simulink model "quadrotor"  (R2020a)
settings: Solver=ode4  StartTime=0.0  StopTime=10  FixedStep=0.01  RelTol=1e-3  EnableMultiTasking=on
settings Model: Creator=fmina  LastModifiedBy=Chenhao
settings DataIOCC: ReturnWorkspaceOutputs=off
settings OptimizationCC: LifeSpan=inf
settings DebuggingCC: SFUnexpectedBacktrackingDiag=warning  SFNoUnconditionalDefaultTransitionDiag=warning  SFExecutionAtInitializationDiag=none  ArithmeticOperatorsInVariantConditions=warning
settings SFSimCC: SimUseLocalCustomCode=off  CustomCodeUndefinedFunction=UseInterfaceOnly
settings RTWCC: RTWUseLocalCustomCode=off
settings CodeAppCC: StateflowObjectComments=on
settings GRTTargetCC: TargetLangStandard=C89/C90 (ANSI)
settings ConfigComp: CovMetricSettings=dw  CovHtmlReporting=on  CovSaveCumulativeToWorkspaceVar=on  CovSaveSingleToWorkspaceVar=on  CovExternalEMLEnable=off

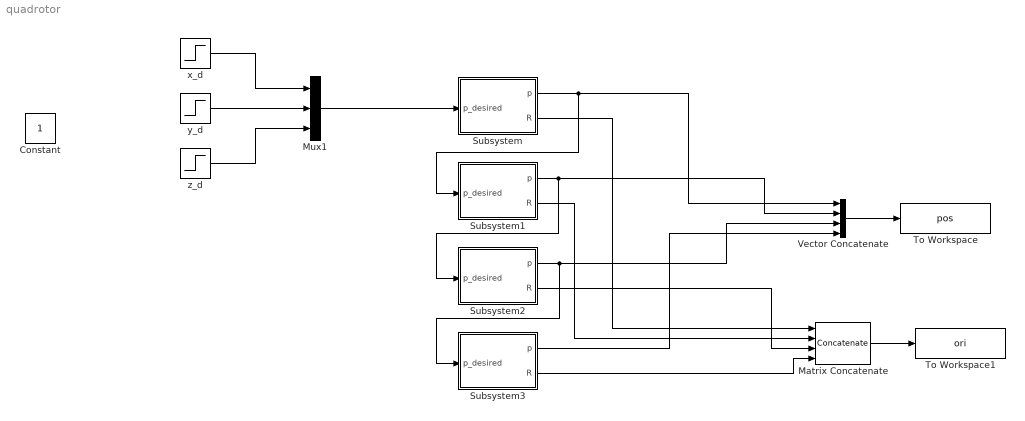
== system quadrotor ==
  Matrix Concatenate : Concatenate  NumInputs=4  Mode=Multidimensional array  ConcatenateDimension=2
  Mux1 : Mux  Inputs=3
  Subsystem : Subsystem
  Subsystem1 : Subsystem
  Subsystem2 : Subsystem
  Subsystem3 : Subsystem
  To Workspace : ToWorkspace  VariableName=pos  SaveFormat=Timeseries  SampleTime=-1
  To Workspace1 : ToWorkspace  VariableName=ori  SaveFormat=Timeseries  SampleTime=-1
  Vector Concatenate : Concatenate  NumInputs=4
  x_d : Step  After=0  SampleTime=0
  y_d : Step  After=0  SampleTime=0
  z_d : Step  Time=0  After=-2  SampleTime=0
  Constant : Constant  IOType=siggen
  wires:
  Mux1/1 -> Subsystem/1(p_desired)
  z_d/1 -> Mux1/3
  y_d/1 -> Mux1/2
  x_d/1 -> Mux1/1
  Vector Concatenate/1 -> To Workspace/1
  Matrix Concatenate/1 -> To Workspace1/1
  Subsystem/1(p) -> Subsystem1/1(p_desired), Vector Concatenate/1
  Subsystem/2(R) -> Matrix Concatenate/1
  Subsystem1/1(p) -> Subsystem2/1(p_desired), Vector Concatenate/2
  Subsystem2/1(p) -> Subsystem3/1(p_desired), Vector Concatenate/3
  Subsystem3/1(p) -> Vector Concatenate/4
  Subsystem1/2(R) -> Matrix Concatenate/2
  Subsystem2/2(R) -> Matrix Concatenate/3
  Subsystem3/2(R) -> Matrix Concatenate/4

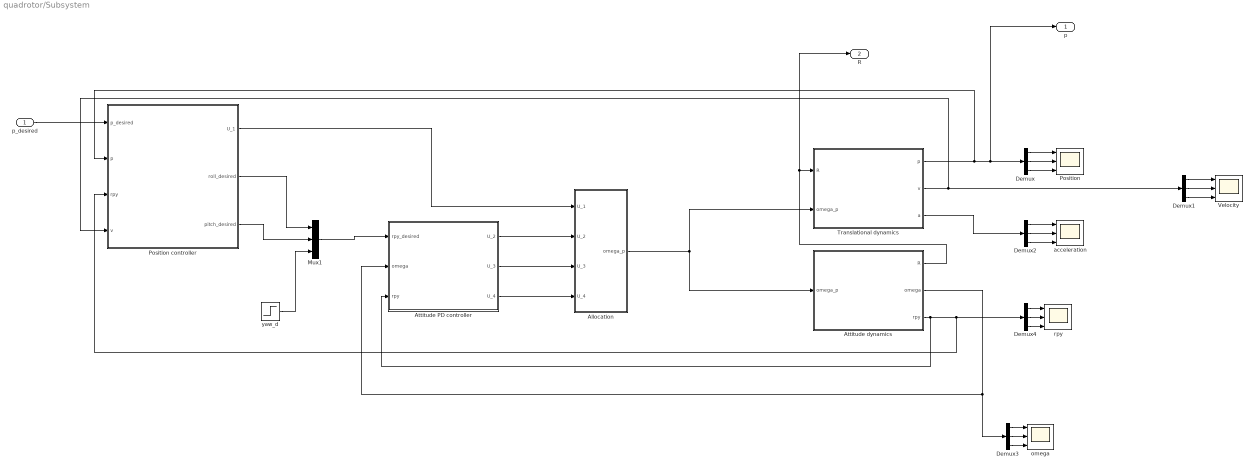
== system quadrotor/Subsystem ==
  p_desired : Inport
  Allocation : Subsystem
  Attitude PD controller : Subsystem
  Attitude dynamics : Subsystem
  Demux{,1..4} (5 alike) : Demux  Outputs=3
  Mux1 : Mux  Inputs=3
  Position : Scope  NumInputPorts=3
  Position controller : Subsystem
  Translational dynamics : Subsystem
  Velocity : Scope  NumInputPorts=3
  acceleration : Scope  NumInputPorts=3
  omega : Scope  NumInputPorts=3
  rpy : Scope  NumInputPorts=3
  yaw_d : Step  After=0  SampleTime=0
  p : Outport  VectorParamsAs1DForOutWhenUnconnected=off
  R : Outport  Port=2  VectorParamsAs1DForOutWhenUnconnected=off
  wires:
  Demux1/3 -> Velocity/3
  Attitude dynamics/2(omega) -> Demux3/1, Attitude PD controller/2("omega ")
  Attitude dynamics/3(rpy) -> Attitude PD controller/3(rpy), Position controller/3(rpy), Demux4/1
  Demux/3 -> Position/3
  Demux4/2 -> rpy/2
  Attitude PD controller/1(U_2) -> Allocation/2(U_2)
  Allocation/1(omega_p) -> Attitude dynamics/1(omega_p), Translational dynamics/2(omega_p)
  Demux3/3 -> omega/3
  Translational dynamics/1(p) -> Position controller/2(p), p/1, Demux/1
  Translational dynamics/3(a) -> Demux2/1
  Attitude PD controller/3(U_4) -> Allocation/4(U_4)
  Demux/1 -> Position/1
  Demux2/3 -> acceleration/3
  yaw_d/1 -> Mux1/3
  Position controller/1(U_1) -> Allocation/1(U_1)
  Translational dynamics/2(v) -> Position controller/4(v), Demux1/1
  Attitude dynamics/1(R) -> R/1, Translational dynamics/1(R)
  Demux/2 -> Position/2
  Position controller/3(pitch_desired) -> Mux1/2
  Mux1/1 -> Attitude PD controller/1(rpy_desired)
  Attitude PD controller/2(U_3) -> Allocation/3(U_3)
  Position controller/2(roll_desired) -> Mux1/1
  Demux1/2 -> Velocity/2
  Demux2/1 -> acceleration/1
  Demux3/2 -> omega/2
  Demux3/1 -> omega/1
  Demux1/1 -> Velocity/1
  Demux4/3 -> rpy/3
  Demux2/2 -> acceleration/2
  Demux4/1 -> rpy/1
  p_desired/1 -> Position controller/1(p_desired)

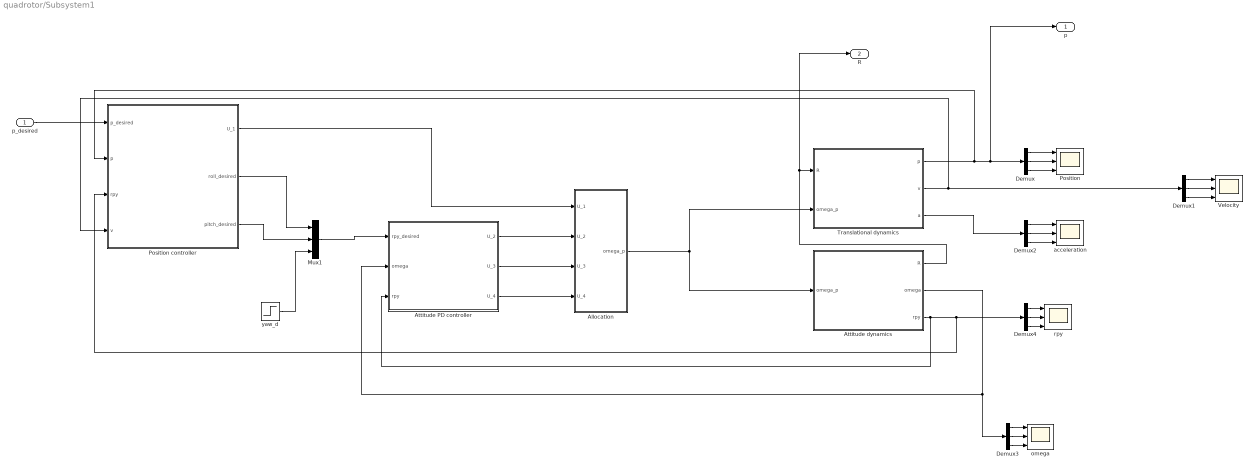
== system quadrotor/Subsystem1 ==
  p_desired : Inport
  Allocation : Subsystem
  Attitude PD controller : Subsystem
  Attitude dynamics : Subsystem
  Demux{,1..4} (5 alike) : Demux  Outputs=3
  Mux1 : Mux  Inputs=3
  Position : Scope  NumInputPorts=3
  Position controller : Subsystem
  Translational dynamics : Subsystem
  Velocity : Scope  NumInputPorts=3
  acceleration : Scope  NumInputPorts=3
  omega : Scope  NumInputPorts=3
  rpy : Scope  NumInputPorts=3
  yaw_d : Step  After=0  SampleTime=0
  p : Outport  VectorParamsAs1DForOutWhenUnconnected=off
  R : Outport  Port=2  VectorParamsAs1DForOutWhenUnconnected=off
  wires:
  Demux1/3 -> Velocity/3
  Attitude dynamics/2(omega) -> Demux3/1, Attitude PD controller/2("omega ")
  Attitude dynamics/3(rpy) -> Attitude PD controller/3(rpy), Position controller/3(rpy), Demux4/1
  Demux/3 -> Position/3
  Demux4/2 -> rpy/2
  Attitude PD controller/1(U_2) -> Allocation/2(U_2)
  Allocation/1(omega_p) -> Attitude dynamics/1(omega_p), Translational dynamics/2(omega_p)
  Demux3/3 -> omega/3
  Translational dynamics/1(p) -> Position controller/2(p), p/1, Demux/1
  Translational dynamics/3(a) -> Demux2/1
  Attitude PD controller/3(U_4) -> Allocation/4(U_4)
  Demux/1 -> Position/1
  Demux2/3 -> acceleration/3
  yaw_d/1 -> Mux1/3
  Position controller/1(U_1) -> Allocation/1(U_1)
  Translational dynamics/2(v) -> Position controller/4(v), Demux1/1
  Attitude dynamics/1(R) -> R/1, Translational dynamics/1(R)
  Demux/2 -> Position/2
  Position controller/3(pitch_desired) -> Mux1/2
  Mux1/1 -> Attitude PD controller/1(rpy_desired)
  Attitude PD controller/2(U_3) -> Allocation/3(U_3)
  Position controller/2(roll_desired) -> Mux1/1
  Demux1/2 -> Velocity/2
  Demux2/1 -> acceleration/1
  Demux3/2 -> omega/2
  Demux3/1 -> omega/1
  Demux1/1 -> Velocity/1
  Demux4/3 -> rpy/3
  Demux2/2 -> acceleration/2
  Demux4/1 -> rpy/1
  p_desired/1 -> Position controller/1(p_desired)

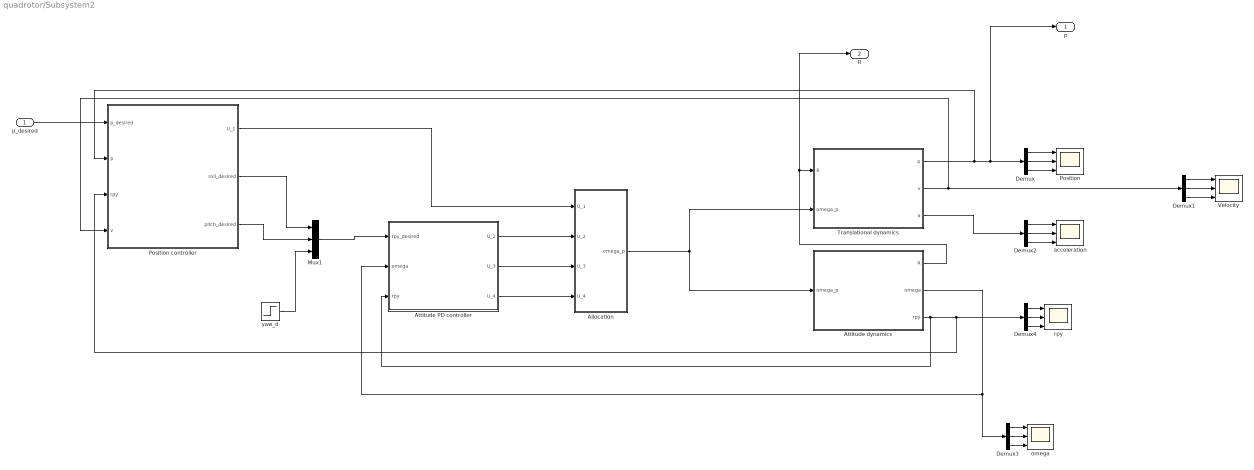
== system quadrotor/Subsystem2 ==
  p_desired : Inport
  Allocation : Subsystem
  Attitude PD controller : Subsystem
  Attitude dynamics : Subsystem
  Demux{,1..4} (5 alike) : Demux  Outputs=3
  Mux1 : Mux  Inputs=3
  Position : Scope  NumInputPorts=3
  Position controller : Subsystem
  Translational dynamics : Subsystem
  Velocity : Scope  NumInputPorts=3
  acceleration : Scope  NumInputPorts=3
  omega : Scope  NumInputPorts=3
  rpy : Scope  NumInputPorts=3
  yaw_d : Step  After=0  SampleTime=0
  p : Outport  VectorParamsAs1DForOutWhenUnconnected=off
  R : Outport  Port=2  VectorParamsAs1DForOutWhenUnconnected=off
  wires:
  Demux1/3 -> Velocity/3
  Attitude dynamics/2(omega) -> Demux3/1, Attitude PD controller/2("omega ")
  Attitude dynamics/3(rpy) -> Attitude PD controller/3(rpy), Position controller/3(rpy), Demux4/1
  Demux/3 -> Position/3
  Demux4/2 -> rpy/2
  Attitude PD controller/1(U_2) -> Allocation/2(U_2)
  Allocation/1(omega_p) -> Attitude dynamics/1(omega_p), Translational dynamics/2(omega_p)
  Demux3/3 -> omega/3
  Translational dynamics/1(p) -> Position controller/2(p), p/1, Demux/1
  Translational dynamics/3(a) -> Demux2/1
  Attitude PD controller/3(U_4) -> Allocation/4(U_4)
  Demux/1 -> Position/1
  Demux2/3 -> acceleration/3
  yaw_d/1 -> Mux1/3
  Position controller/1(U_1) -> Allocation/1(U_1)
  Translational dynamics/2(v) -> Position controller/4(v), Demux1/1
  Attitude dynamics/1(R) -> R/1, Translational dynamics/1(R)
  Demux/2 -> Position/2
  Position controller/3(pitch_desired) -> Mux1/2
  Mux1/1 -> Attitude PD controller/1(rpy_desired)
  Attitude PD controller/2(U_3) -> Allocation/3(U_3)
  Position controller/2(roll_desired) -> Mux1/1
  Demux1/2 -> Velocity/2
  Demux2/1 -> acceleration/1
  Demux3/2 -> omega/2
  Demux3/1 -> omega/1
  Demux1/1 -> Velocity/1
  Demux4/3 -> rpy/3
  Demux2/2 -> acceleration/2
  Demux4/1 -> rpy/1
  p_desired/1 -> Position controller/1(p_desired)

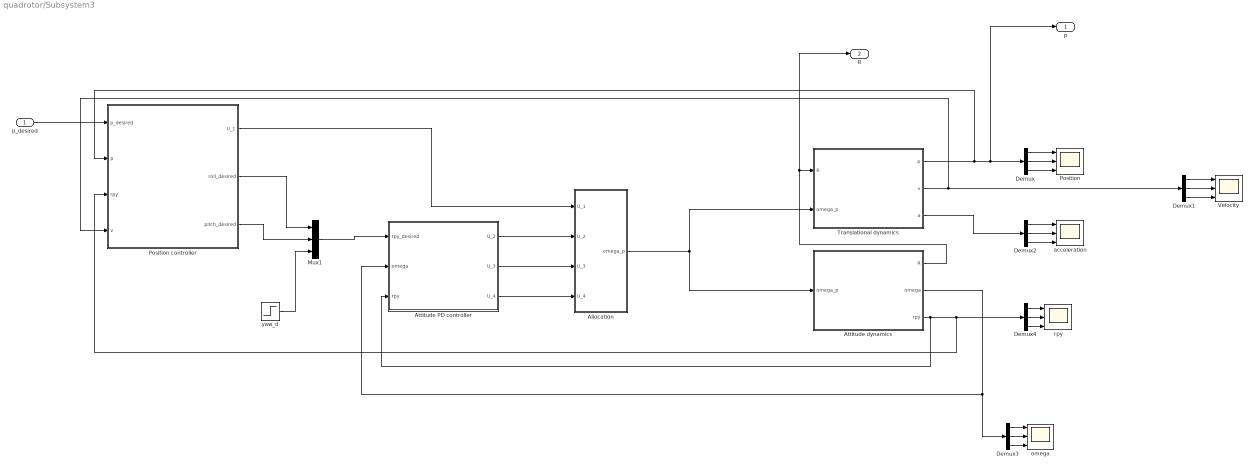
== system quadrotor/Subsystem3 ==
  p_desired : Inport
  Allocation : Subsystem
  Attitude PD controller : Subsystem
  Attitude dynamics : Subsystem
  Demux{,1..4} (5 alike) : Demux  Outputs=3
  Mux1 : Mux  Inputs=3
  Position : Scope  NumInputPorts=3
  Position controller : Subsystem
  Translational dynamics : Subsystem
  Velocity : Scope  NumInputPorts=3
  acceleration : Scope  NumInputPorts=3
  omega : Scope  NumInputPorts=3
  rpy : Scope  NumInputPorts=3
  yaw_d : Step  After=0  SampleTime=0
  p : Outport  VectorParamsAs1DForOutWhenUnconnected=off
  R : Outport  Port=2  VectorParamsAs1DForOutWhenUnconnected=off
  wires:
  Demux1/3 -> Velocity/3
  Attitude dynamics/2(omega) -> Demux3/1, Attitude PD controller/2("omega ")
  Attitude dynamics/3(rpy) -> Attitude PD controller/3(rpy), Position controller/3(rpy), Demux4/1
  Demux/3 -> Position/3
  Demux4/2 -> rpy/2
  Attitude PD controller/1(U_2) -> Allocation/2(U_2)
  Allocation/1(omega_p) -> Attitude dynamics/1(omega_p), Translational dynamics/2(omega_p)
  Demux3/3 -> omega/3
  Translational dynamics/1(p) -> Position controller/2(p), p/1, Demux/1
  Translational dynamics/3(a) -> Demux2/1
  Attitude PD controller/3(U_4) -> Allocation/4(U_4)
  Demux/1 -> Position/1
  Demux2/3 -> acceleration/3
  yaw_d/1 -> Mux1/3
  Position controller/1(U_1) -> Allocation/1(U_1)
  Translational dynamics/2(v) -> Position controller/4(v), Demux1/1
  Attitude dynamics/1(R) -> R/1, Translational dynamics/1(R)
  Demux/2 -> Position/2
  Position controller/3(pitch_desired) -> Mux1/2
  Mux1/1 -> Attitude PD controller/1(rpy_desired)
  Attitude PD controller/2(U_3) -> Allocation/3(U_3)
  Position controller/2(roll_desired) -> Mux1/1
  Demux1/2 -> Velocity/2
  Demux2/1 -> acceleration/1
  Demux3/2 -> omega/2
  Demux3/1 -> omega/1
  Demux1/1 -> Velocity/1
  Demux4/3 -> rpy/3
  Demux2/2 -> acceleration/2
  Demux4/1 -> rpy/1
  p_desired/1 -> Position controller/1(p_desired)

== system quadrotor/Subsystem/Allocation ==
  U_1 : Inport
  U_2 : Inport  Port=2
  U_3 : Inport  Port=3
  U_4 : Inport  Port=4
  Control allocation : MATLAB Function  TreatAsAtomicUnit=on
  omega_p : Outport  PortDimensions=[4,1]  VectorParamsAs1DForOutWhenUnconnected=off
  wires:
  U_1/1 -> Control allocation/1(U_1)
  Control allocation/1(omega_p) -> omega_p/1
  U_4/1 -> Control allocation/4(U_4)
  U_2/1 -> Control allocation/2(U_2)
  U_3/1 -> Control allocation/3(U_3)

== system quadrotor/Subsystem/Attitude PD controller ==
  rpy_desired : Inport
  "omega " : Inport  Port=2
  rpy : Inport  Port=3
  Demux : Demux  Outputs=3
  PD_attitude_controller_eqn : MATLAB Function  TreatAsAtomicUnit=on
  U_2 : Outport  VectorParamsAs1DForOutWhenUnconnected=off
  U_3 : Outport  Port=2  VectorParamsAs1DForOutWhenUnconnected=off
  U_4 : Outport  Port=3  VectorParamsAs1DForOutWhenUnconnected=off
  wires:
  rpy_desired/1 -> PD_attitude_controller_eqn/1(rpy_desired)
  rpy/1 -> PD_attitude_controller_eqn/2(rpy)
  "omega "/1 -> PD_attitude_controller_eqn/3(omega)
  PD_attitude_controller_eqn/1(U_2_3_4) -> Demux/1
  Demux/1 -> U_2/1
  Demux/2 -> U_3/1
  Demux/3 -> U_4/1

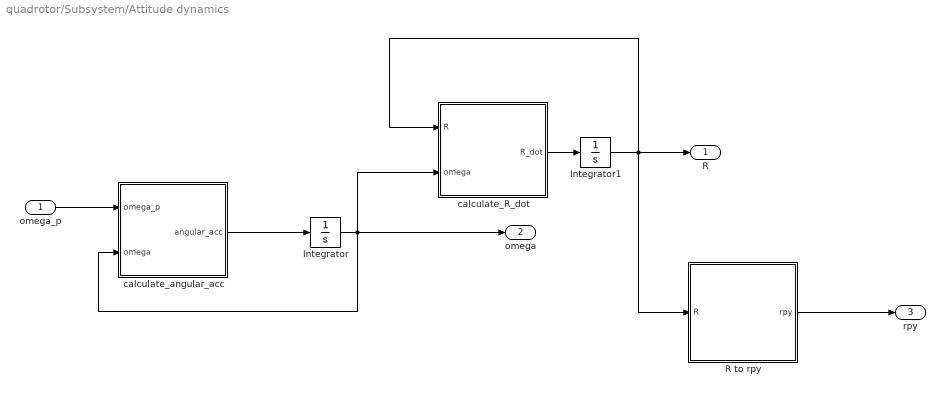
== system quadrotor/Subsystem/Attitude dynamics ==
  omega_p : Inport
  Integrator : Integrator  InitialCondition=zeros(3,1)
  Integrator1 : Integrator  InitialCondition=eye(3)
  R to rpy : MATLAB Function  TreatAsAtomicUnit=on
  calculate_R_dot : MATLAB Function  TreatAsAtomicUnit=on
  calculate_angular_acc : MATLAB Function  TreatAsAtomicUnit=on
  R : Outport  VectorParamsAs1DForOutWhenUnconnected=off
  omega : Outport  Port=2  VectorParamsAs1DForOutWhenUnconnected=off
  rpy : Outport  Port=3  VectorParamsAs1DForOutWhenUnconnected=off
  wires:
  omega_p/1 -> calculate_angular_acc/1(omega_p)
  calculate_angular_acc/1(angular_acc) -> Integrator/1
  Integrator/1 -> calculate_R_dot/2(omega), calculate_angular_acc/2(omega), omega/1
  calculate_R_dot/1(R_dot) -> Integrator1/1
  R to rpy/1(rpy) -> rpy/1
  Integrator1/1 -> R to rpy/1(R), calculate_R_dot/1(R), R/1

== system quadrotor/Subsystem/Position controller ==
  p_desired : Inport
  p : Inport  Port=2
  rpy : Inport  Port=3
  v : Inport  Port=4
  PD_position_controller_eqn : MATLAB Function  TreatAsAtomicUnit=on
  U_1 : Outport  VectorParamsAs1DForOutWhenUnconnected=off
  roll_desired : Outport  Port=2  VectorParamsAs1DForOutWhenUnconnected=off
  pitch_desired : Outport  Port=3  VectorParamsAs1DForOutWhenUnconnected=off
  wires:
  p_desired/1 -> PD_position_controller_eqn/1(p_d)
  v/1 -> PD_position_controller_eqn/4(v)
  PD_position_controller_eqn/1(U_1) -> U_1/1
  p/1 -> PD_position_controller_eqn/2(p)
  rpy/1 -> PD_position_controller_eqn/3(rpy)
  PD_position_controller_eqn/2(roll_d) -> roll_desired/1
  PD_position_controller_eqn/3(pitch_d) -> pitch_desired/1

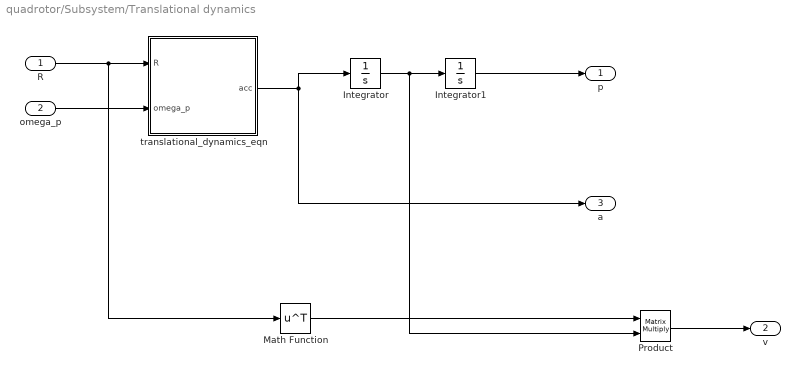
== system quadrotor/Subsystem/Translational dynamics ==
  R : Inport
  omega_p : Inport  Port=2
  Integrator : Integrator
  Integrator1 : Integrator  InitialCondition=[-2 2 0]
  Math Function : Math  Operator=transpose  SignedPower=on  SaturateOnIntegerOverflow=on
  Product : Product  Multiplication=Matrix(*)
  translational_dynamics_eqn : MATLAB Function  TreatAsAtomicUnit=on
  p : Outport  VectorParamsAs1DForOutWhenUnconnected=off
  v : Outport  Port=2  VectorParamsAs1DForOutWhenUnconnected=off
  a : Outport  Port=3  VectorParamsAs1DForOutWhenUnconnected=off
  wires:
  translational_dynamics_eqn/1(acc) -> Integrator/1, a/1
  Integrator/1 -> Product/2, Integrator1/1
  Integrator1/1 -> p/1
  omega_p/1 -> translational_dynamics_eqn/2(omega_p)
  R/1 -> translational_dynamics_eqn/1(R), Math Function/1
  Math Function/1 -> Product/1
  Product/1 -> v/1

== system quadrotor/Subsystem1/Allocation ==
  U_1 : Inport
  U_2 : Inport  Port=2
  U_3 : Inport  Port=3
  U_4 : Inport  Port=4
  Control allocation : MATLAB Function  TreatAsAtomicUnit=on
  omega_p : Outport  PortDimensions=[4,1]  VectorParamsAs1DForOutWhenUnconnected=off
  wires:
  U_1/1 -> Control allocation/1(U_1)
  Control allocation/1(omega_p) -> omega_p/1
  U_4/1 -> Control allocation/4(U_4)
  U_2/1 -> Control allocation/2(U_2)
  U_3/1 -> Control allocation/3(U_3)

== system quadrotor/Subsystem1/Attitude PD controller ==
  rpy_desired : Inport
  "omega " : Inport  Port=2
  rpy : Inport  Port=3
  Demux : Demux  Outputs=3
  PD_attitude_controller_eqn : MATLAB Function  TreatAsAtomicUnit=on
  U_2 : Outport  VectorParamsAs1DForOutWhenUnconnected=off
  U_3 : Outport  Port=2  VectorParamsAs1DForOutWhenUnconnected=off
  U_4 : Outport  Port=3  VectorParamsAs1DForOutWhenUnconnected=off
  wires:
  rpy_desired/1 -> PD_attitude_controller_eqn/1(rpy_desired)
  rpy/1 -> PD_attitude_controller_eqn/2(rpy)
  "omega "/1 -> PD_attitude_controller_eqn/3(omega)
  PD_attitude_controller_eqn/1(U_2_3_4) -> Demux/1
  Demux/1 -> U_2/1
  Demux/2 -> U_3/1
  Demux/3 -> U_4/1

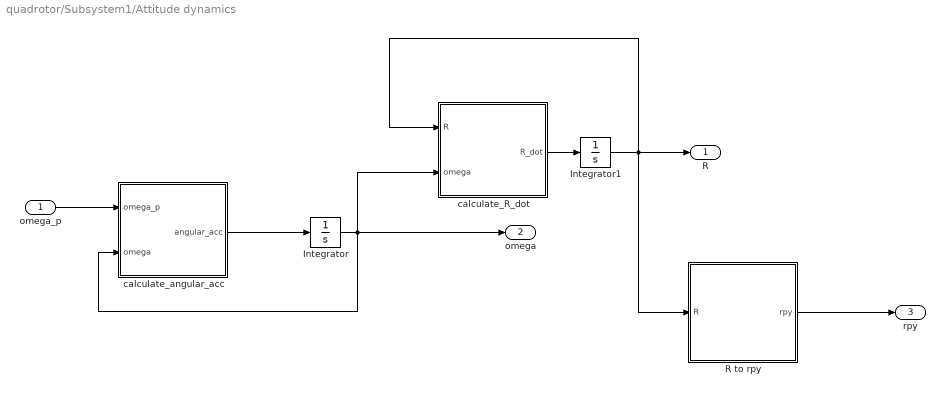
== system quadrotor/Subsystem1/Attitude dynamics ==
  omega_p : Inport
  Integrator : Integrator  InitialCondition=zeros(3,1)
  Integrator1 : Integrator  InitialCondition=eye(3)
  R to rpy : MATLAB Function  TreatAsAtomicUnit=on
  calculate_R_dot : MATLAB Function  TreatAsAtomicUnit=on
  calculate_angular_acc : MATLAB Function  TreatAsAtomicUnit=on
  R : Outport  VectorParamsAs1DForOutWhenUnconnected=off
  omega : Outport  Port=2  VectorParamsAs1DForOutWhenUnconnected=off
  rpy : Outport  Port=3  VectorParamsAs1DForOutWhenUnconnected=off
  wires:
  omega_p/1 -> calculate_angular_acc/1(omega_p)
  calculate_angular_acc/1(angular_acc) -> Integrator/1
  Integrator/1 -> calculate_R_dot/2(omega), calculate_angular_acc/2(omega), omega/1
  calculate_R_dot/1(R_dot) -> Integrator1/1
  R to rpy/1(rpy) -> rpy/1
  Integrator1/1 -> R to rpy/1(R), calculate_R_dot/1(R), R/1

== system quadrotor/Subsystem1/Position controller ==
  p_desired : Inport
  p : Inport  Port=2
  rpy : Inport  Port=3
  v : Inport  Port=4
  PD_position_controller_eqn : MATLAB Function  TreatAsAtomicUnit=on
  U_1 : Outport  VectorParamsAs1DForOutWhenUnconnected=off
  roll_desired : Outport  Port=2  VectorParamsAs1DForOutWhenUnconnected=off
  pitch_desired : Outport  Port=3  VectorParamsAs1DForOutWhenUnconnected=off
  wires:
  p_desired/1 -> PD_position_controller_eqn/1(p_d)
  v/1 -> PD_position_controller_eqn/4(v)
  PD_position_controller_eqn/1(U_1) -> U_1/1
  p/1 -> PD_position_controller_eqn/2(p)
  rpy/1 -> PD_position_controller_eqn/3(rpy)
  PD_position_controller_eqn/2(roll_d) -> roll_desired/1
  PD_position_controller_eqn/3(pitch_d) -> pitch_desired/1

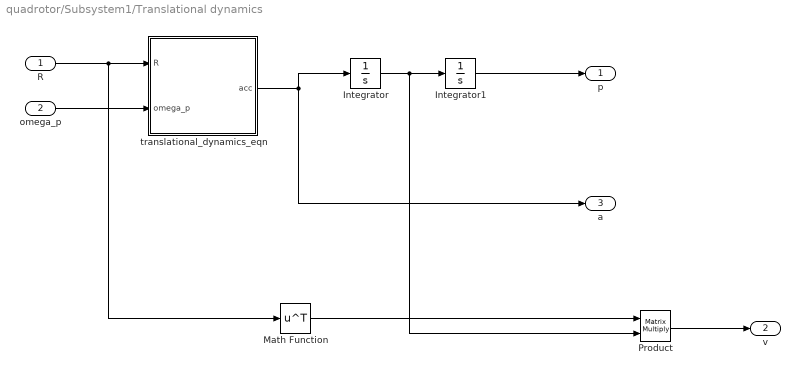
== system quadrotor/Subsystem1/Translational dynamics ==
  R : Inport
  omega_p : Inport  Port=2
  Integrator : Integrator
  Integrator1 : Integrator  InitialCondition=[-2 -2 0]
  Math Function : Math  Operator=transpose  SignedPower=on  SaturateOnIntegerOverflow=on
  Product : Product  Multiplication=Matrix(*)
  translational_dynamics_eqn : MATLAB Function  TreatAsAtomicUnit=on
  p : Outport  VectorParamsAs1DForOutWhenUnconnected=off
  v : Outport  Port=2  VectorParamsAs1DForOutWhenUnconnected=off
  a : Outport  Port=3  VectorParamsAs1DForOutWhenUnconnected=off
  wires:
  translational_dynamics_eqn/1(acc) -> Integrator/1, a/1
  Integrator/1 -> Product/2, Integrator1/1
  Integrator1/1 -> p/1
  omega_p/1 -> translational_dynamics_eqn/2(omega_p)
  R/1 -> translational_dynamics_eqn/1(R), Math Function/1
  Math Function/1 -> Product/1
  Product/1 -> v/1

== system quadrotor/Subsystem2/Allocation ==
  U_1 : Inport
  U_2 : Inport  Port=2
  U_3 : Inport  Port=3
  U_4 : Inport  Port=4
  Control allocation : MATLAB Function  TreatAsAtomicUnit=on
  omega_p : Outport  PortDimensions=[4,1]  VectorParamsAs1DForOutWhenUnconnected=off
  wires:
  U_1/1 -> Control allocation/1(U_1)
  Control allocation/1(omega_p) -> omega_p/1
  U_4/1 -> Control allocation/4(U_4)
  U_2/1 -> Control allocation/2(U_2)
  U_3/1 -> Control allocation/3(U_3)

== system quadrotor/Subsystem2/Attitude PD controller ==
  rpy_desired : Inport
  "omega " : Inport  Port=2
  rpy : Inport  Port=3
  Demux : Demux  Outputs=3
  PD_attitude_controller_eqn : MATLAB Function  TreatAsAtomicUnit=on
  U_2 : Outport  VectorParamsAs1DForOutWhenUnconnected=off
  U_3 : Outport  Port=2  VectorParamsAs1DForOutWhenUnconnected=off
  U_4 : Outport  Port=3  VectorParamsAs1DForOutWhenUnconnected=off
  wires:
  rpy_desired/1 -> PD_attitude_controller_eqn/1(rpy_desired)
  rpy/1 -> PD_attitude_controller_eqn/2(rpy)
  "omega "/1 -> PD_attitude_controller_eqn/3(omega)
  PD_attitude_controller_eqn/1(U_2_3_4) -> Demux/1
  Demux/1 -> U_2/1
  Demux/2 -> U_3/1
  Demux/3 -> U_4/1

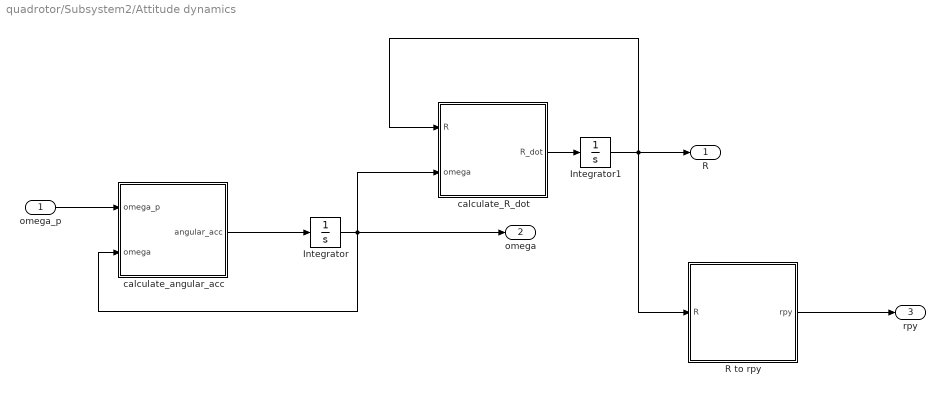
== system quadrotor/Subsystem2/Attitude dynamics ==
  omega_p : Inport
  Integrator : Integrator  InitialCondition=zeros(3,1)
  Integrator1 : Integrator  InitialCondition=eye(3)
  R to rpy : MATLAB Function  TreatAsAtomicUnit=on
  calculate_R_dot : MATLAB Function  TreatAsAtomicUnit=on
  calculate_angular_acc : MATLAB Function  TreatAsAtomicUnit=on
  R : Outport  VectorParamsAs1DForOutWhenUnconnected=off
  omega : Outport  Port=2  VectorParamsAs1DForOutWhenUnconnected=off
  rpy : Outport  Port=3  VectorParamsAs1DForOutWhenUnconnected=off
  wires:
  omega_p/1 -> calculate_angular_acc/1(omega_p)
  calculate_angular_acc/1(angular_acc) -> Integrator/1
  Integrator/1 -> calculate_R_dot/2(omega), calculate_angular_acc/2(omega), omega/1
  calculate_R_dot/1(R_dot) -> Integrator1/1
  R to rpy/1(rpy) -> rpy/1
  Integrator1/1 -> R to rpy/1(R), calculate_R_dot/1(R), R/1

== system quadrotor/Subsystem2/Position controller ==
  p_desired : Inport
  p : Inport  Port=2
  rpy : Inport  Port=3
  v : Inport  Port=4
  PD_position_controller_eqn : MATLAB Function  TreatAsAtomicUnit=on
  U_1 : Outport  VectorParamsAs1DForOutWhenUnconnected=off
  roll_desired : Outport  Port=2  VectorParamsAs1DForOutWhenUnconnected=off
  pitch_desired : Outport  Port=3  VectorParamsAs1DForOutWhenUnconnected=off
  wires:
  p_desired/1 -> PD_position_controller_eqn/1(p_d)
  v/1 -> PD_position_controller_eqn/4(v)
  PD_position_controller_eqn/1(U_1) -> U_1/1
  p/1 -> PD_position_controller_eqn/2(p)
  rpy/1 -> PD_position_controller_eqn/3(rpy)
  PD_position_controller_eqn/2(roll_d) -> roll_desired/1
  PD_position_controller_eqn/3(pitch_d) -> pitch_desired/1

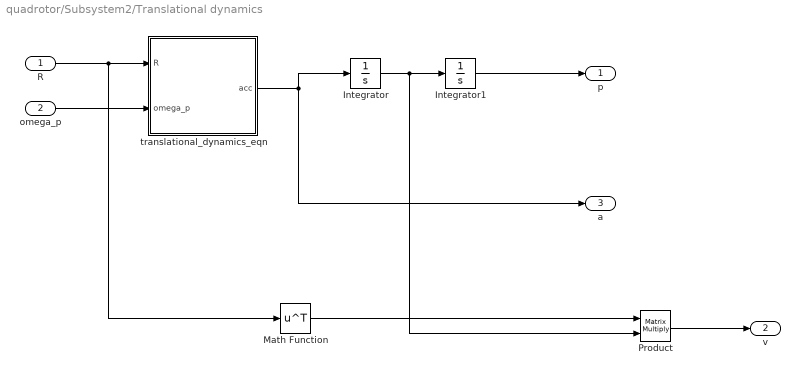
== system quadrotor/Subsystem2/Translational dynamics ==
  R : Inport
  omega_p : Inport  Port=2
  Integrator : Integrator
  Integrator1 : Integrator  InitialCondition=[2 -2 0]
  Math Function : Math  Operator=transpose  SignedPower=on  SaturateOnIntegerOverflow=on
  Product : Product  Multiplication=Matrix(*)
  translational_dynamics_eqn : MATLAB Function  TreatAsAtomicUnit=on
  p : Outport  VectorParamsAs1DForOutWhenUnconnected=off
  v : Outport  Port=2  VectorParamsAs1DForOutWhenUnconnected=off
  a : Outport  Port=3  VectorParamsAs1DForOutWhenUnconnected=off
  wires:
  translational_dynamics_eqn/1(acc) -> Integrator/1, a/1
  Integrator/1 -> Product/2, Integrator1/1
  Integrator1/1 -> p/1
  omega_p/1 -> translational_dynamics_eqn/2(omega_p)
  R/1 -> translational_dynamics_eqn/1(R), Math Function/1
  Math Function/1 -> Product/1
  Product/1 -> v/1

== system quadrotor/Subsystem3/Allocation ==
  U_1 : Inport
  U_2 : Inport  Port=2
  U_3 : Inport  Port=3
  U_4 : Inport  Port=4
  Control allocation : MATLAB Function  TreatAsAtomicUnit=on
  omega_p : Outport  PortDimensions=[4,1]  VectorParamsAs1DForOutWhenUnconnected=off
  wires:
  U_1/1 -> Control allocation/1(U_1)
  Control allocation/1(omega_p) -> omega_p/1
  U_4/1 -> Control allocation/4(U_4)
  U_2/1 -> Control allocation/2(U_2)
  U_3/1 -> Control allocation/3(U_3)

== system quadrotor/Subsystem3/Attitude PD controller ==
  rpy_desired : Inport
  "omega " : Inport  Port=2
  rpy : Inport  Port=3
  Demux : Demux  Outputs=3
  PD_attitude_controller_eqn : MATLAB Function  TreatAsAtomicUnit=on
  U_2 : Outport  VectorParamsAs1DForOutWhenUnconnected=off
  U_3 : Outport  Port=2  VectorParamsAs1DForOutWhenUnconnected=off
  U_4 : Outport  Port=3  VectorParamsAs1DForOutWhenUnconnected=off
  wires:
  rpy_desired/1 -> PD_attitude_controller_eqn/1(rpy_desired)
  rpy/1 -> PD_attitude_controller_eqn/2(rpy)
  "omega "/1 -> PD_attitude_controller_eqn/3(omega)
  PD_attitude_controller_eqn/1(U_2_3_4) -> Demux/1
  Demux/1 -> U_2/1
  Demux/2 -> U_3/1
  Demux/3 -> U_4/1

== system quadrotor/Subsystem3/Attitude dynamics ==
  omega_p : Inport
  Integrator : Integrator  InitialCondition=zeros(3,1)
  Integrator1 : Integrator  InitialCondition=eye(3)
  R to rpy : MATLAB Function  TreatAsAtomicUnit=on
  calculate_R_dot : MATLAB Function  TreatAsAtomicUnit=on
  calculate_angular_acc : MATLAB Function  TreatAsAtomicUnit=on
  R : Outport  VectorParamsAs1DForOutWhenUnconnected=off
  omega : Outport  Port=2  VectorParamsAs1DForOutWhenUnconnected=off
  rpy : Outport  Port=3  VectorParamsAs1DForOutWhenUnconnected=off
  wires:
  omega_p/1 -> calculate_angular_acc/1(omega_p)
  calculate_angular_acc/1(angular_acc) -> Integrator/1
  Integrator/1 -> calculate_R_dot/2(omega), calculate_angular_acc/2(omega), omega/1
  calculate_R_dot/1(R_dot) -> Integrator1/1
  R to rpy/1(rpy) -> rpy/1
  Integrator1/1 -> R to rpy/1(R), calculate_R_dot/1(R), R/1

== system quadrotor/Subsystem3/Position controller ==
  p_desired : Inport
  p : Inport  Port=2
  rpy : Inport  Port=3
  v : Inport  Port=4
  PD_position_controller_eqn : MATLAB Function  TreatAsAtomicUnit=on
  U_1 : Outport  VectorParamsAs1DForOutWhenUnconnected=off
  roll_desired : Outport  Port=2  VectorParamsAs1DForOutWhenUnconnected=off
  pitch_desired : Outport  Port=3  VectorParamsAs1DForOutWhenUnconnected=off
  wires:
  p_desired/1 -> PD_position_controller_eqn/1(p_d)
  v/1 -> PD_position_controller_eqn/4(v)
  PD_position_controller_eqn/1(U_1) -> U_1/1
  p/1 -> PD_position_controller_eqn/2(p)
  rpy/1 -> PD_position_controller_eqn/3(rpy)
  PD_position_controller_eqn/2(roll_d) -> roll_desired/1
  PD_position_controller_eqn/3(pitch_d) -> pitch_desired/1

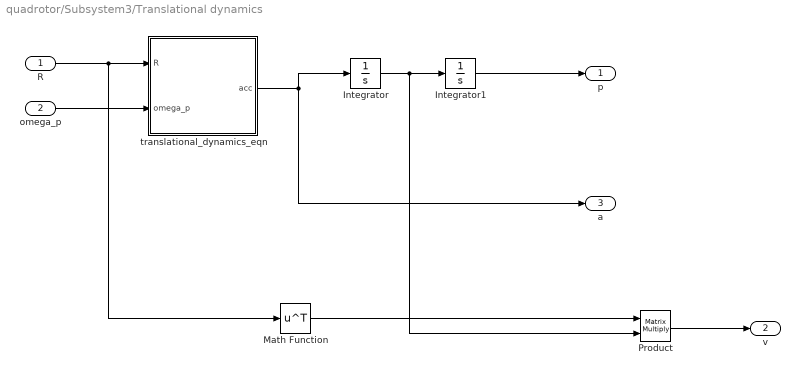
== system quadrotor/Subsystem3/Translational dynamics ==
  R : Inport
  omega_p : Inport  Port=2
  Integrator : Integrator
  Integrator1 : Integrator  InitialCondition=[2 2 0]
  Math Function : Math  Operator=transpose  SignedPower=on  SaturateOnIntegerOverflow=on
  Product : Product  Multiplication=Matrix(*)
  translational_dynamics_eqn : MATLAB Function  TreatAsAtomicUnit=on
  p : Outport  VectorParamsAs1DForOutWhenUnconnected=off
  v : Outport  Port=2  VectorParamsAs1DForOutWhenUnconnected=off
  a : Outport  Port=3  VectorParamsAs1DForOutWhenUnconnected=off
  wires:
  translational_dynamics_eqn/1(acc) -> Integrator/1, a/1
  Integrator/1 -> Product/2, Integrator1/1
  Integrator1/1 -> p/1
  omega_p/1 -> translational_dynamics_eqn/2(omega_p)
  R/1 -> translational_dynamics_eqn/1(R), Math Function/1
  Math Function/1 -> Product/1
  Product/1 -> v/1

== matlab function quadrotor/Subsystem1/Attitude dynamics/R to rpy ==
  data: R input; rpy output
function rpy = fcn(R)

%calculate roll pitch yaw from rotation matrix

[U,~,V] = svd(R);
R = U*V';

pitch = asin(-R(3,1));
roll = atan2(R(3,2), R(3,3));
yaw = atan2(R(2,1), R(1,1));

rpy = [roll; pitch; yaw];

== matlab function quadrotor/Subsystem1/Attitude dynamics/calculate_R_dot ==
  data: R input; R_dot output; omega input
function R_dot = fcn(R, omega)

%load parameters
params = parameters();

%normalize R every step to guarantee that R is orthogonal matrix (valid
%rotation)
[U,~,V] = svd(R);
R = U*V';

%Write R_dot = R*skew_omega
R_dot = R*[0 -omega(3) omega(2); omega(3) 0 -omega(1); -omega(2) omega(1) 0];

== matlab function quadrotor/Subsystem1/Attitude dynamics/calculate_angular_acc ==
  data: omega_p input; angular_acc output; omega input
function angular_acc = fcn(omega_p, omega)
%omega_p is the rotational speed of the propellers. This vector must have
%size 4.
%omega is the angular velocity of the MAV expressed in body frame.

%load parameters
%Inertia is found under params.J
params = parameters();


U = params.allocation_matrix * (omega_p.^2);
angular_acc = params.J \ (-cross(omega, params.J * omega) + U(2:4));

== matlab function quadrotor/Subsystem1/Position controller/PD_position_controller_eqn ==
  data: p_d input; p input; rpy input; U_1 output; v input; roll_d output; pitch_d output
function [U_1, roll_d, pitch_d] = fcn(p_d, p, rpy, v)
%load parameters
%controller Kp is found under params.velocity_Kp
params = parameters();

%control error is given by
p_error = p_d - p;
v_error = zeros(3, 1) - v;
%control action U is given by
roll = rpy(1);
pitch = rpy(2);
yaw = rpy(3);

T = -diag(params.position_Kp) * p_error - diag(params.position_Kd) * v_error + [0; 0; params.m * params.g];

T_z = T(3);
U_1 = T_z / (cos(roll) * cos(pitch));
C_E1 = [cos(yaw) -sin(yaw) 0; sin(yaw) cos(yaw) 0; 0 0 1];
a = 1 / norm(T) * C_E1' * T;
roll_d = min(pi/6, max(-pi/6, -asin(a(2))));
pitch_d = min(pi/6, max(-pi/6, atan2(a(1), a(3))));

== matlab function quadrotor/Subsystem1/Translational dynamics/translational_dynamics_eqn ==
  data: R input; acc output; omega_p input
function acc = fcn(R, omega_p)

%load parameters
% to access for instance vehicle mass, use params.m.
% accelerational gravity is under params.g
params = parameters();

U = params.allocation_matrix*(omega_p.^2);

%acceleration is given by:
acc = - R * [0; 0; U(1)] / params.m + [0; 0; params.g];

== matlab function quadrotor/Subsystem2/Allocation/Control allocation ==
  data: U_1 input; omega_p output; U_2 input; U_3 input; U_4 input
function omega_p = fcn(U_1, U_2, U_3, U_4)

%load parameters

params = parameters();

omega_p_sqr = params.pinv_allocation_matrix*[U_1; U_2; U_3; U_4];

%make sure only positive values are allowed.
omega_p_sqr = max(omega_p_sqr, zeros(4,1));

%actual rotors velocities
omega_p = sqrt(omega_p_sqr);

== matlab function quadrotor/Subsystem2/Attitude PD controller/PD_attitude_controller_eqn ==
  data: rpy_desired input; U_2_3_4 output; rpy input; omega input
function U_2_3_4 = fcn(rpy_desired, rpy, omega)

%load parameters
%controller Kp is found under params.attitude_Kp
%controller Kd is found under params.attitude_Kd
params = parameters();

roll = rpy(1);
pitch = rpy(2);
yaw = rpy(3);

%control error is given by
error = rpy_desired-rpy;

% Relation between Tait-Bryan angles and angular velocities
%E_r = ...
E_r = [1 0 -sin(pitch); ...
       0 cos(roll) sin(roll)*cos(pitch);...
       0 -sin(roll) cos(roll)*cos(pitch)];

% rpy_dot = ... (from omega in body frame)
rpy_dot = E_r \ omega; %inv(E_r)*omega;

%control action U_2_3_4 is given by
%U_2_3_4 = ...

U_2_3_4 = diag(params.attitude_Kp)*error - diag(params.attitude_Kd)*rpy_dot;

== matlab function quadrotor/Subsystem2/Attitude dynamics/R to rpy ==
  data: R input; rpy output
function rpy = fcn(R)

%calculate roll pitch yaw from rotation matrix

[U,~,V] = svd(R);
R = U*V';

pitch = asin(-R(3,1));
roll = atan2(R(3,2), R(3,3));
yaw = atan2(R(2,1), R(1,1));

rpy = [roll; pitch; yaw];

== matlab function quadrotor/Subsystem2/Attitude dynamics/calculate_R_dot ==
  data: R input; R_dot output; omega input
function R_dot = fcn(R, omega)

%load parameters
params = parameters();

%normalize R every step to guarantee that R is orthogonal matrix (valid
%rotation)
[U,~,V] = svd(R);
R = U*V';

%Write R_dot = R*skew_omega
R_dot = R*[0 -omega(3) omega(2); omega(3) 0 -omega(1); -omega(2) omega(1) 0];

== matlab function quadrotor/Subsystem2/Attitude dynamics/calculate_angular_acc ==
  data: omega_p input; angular_acc output; omega input
function angular_acc = fcn(omega_p, omega)
%omega_p is the rotational speed of the propellers. This vector must have
%size 4.
%omega is the angular velocity of the MAV expressed in body frame.

%load parameters
%Inertia is found under params.J
params = parameters();


U = params.allocation_matrix * (omega_p.^2);
angular_acc = params.J \ (-cross(omega, params.J * omega) + U(2:4));

== matlab function quadrotor/Subsystem2/Position controller/PD_position_controller_eqn ==
  data: p_d input; p input; rpy input; U_1 output; v input; roll_d output; pitch_d output
function [U_1, roll_d, pitch_d] = fcn(p_d, p, rpy, v)
%load parameters
%controller Kp is found under params.velocity_Kp
params = parameters();

%control error is given by
p_error = p_d - p;
v_error = zeros(3, 1) - v;
%control action U is given by
roll = rpy(1);
pitch = rpy(2);
yaw = rpy(3);

T = -diag(params.position_Kp) * p_error - diag(params.position_Kd) * v_error + [0; 0; params.m * params.g];

T_z = T(3);
U_1 = T_z / (cos(roll) * cos(pitch));
C_E1 = [cos(yaw) -sin(yaw) 0; sin(yaw) cos(yaw) 0; 0 0 1];
a = 1 / norm(T) * C_E1' * T;
roll_d = min(pi/6, max(-pi/6, -asin(a(2))));
pitch_d = min(pi/6, max(-pi/6, atan2(a(1), a(3))));

== matlab function quadrotor/Subsystem2/Translational dynamics/translational_dynamics_eqn ==
  data: R input; acc output; omega_p input
function acc = fcn(R, omega_p)

%load parameters
% to access for instance vehicle mass, use params.m.
% accelerational gravity is under params.g
params = parameters();

U = params.allocation_matrix*(omega_p.^2);

%acceleration is given by:
acc = - R * [0; 0; U(1)] / params.m + [0; 0; params.g];

== matlab function quadrotor/Subsystem3/Allocation/Control allocation ==
  data: U_1 input; omega_p output; U_2 input; U_3 input; U_4 input
function omega_p = fcn(U_1, U_2, U_3, U_4)

%load parameters

params = parameters();

omega_p_sqr = params.pinv_allocation_matrix*[U_1; U_2; U_3; U_4];

%make sure only positive values are allowed.
omega_p_sqr = max(omega_p_sqr, zeros(4,1));

%actual rotors velocities
omega_p = sqrt(omega_p_sqr);

== matlab function quadrotor/Subsystem3/Attitude PD controller/PD_attitude_controller_eqn ==
  data: rpy_desired input; U_2_3_4 output; rpy input; omega input
function U_2_3_4 = fcn(rpy_desired, rpy, omega)

%load parameters
%controller Kp is found under params.attitude_Kp
%controller Kd is found under params.attitude_Kd
params = parameters();

roll = rpy(1);
pitch = rpy(2);
yaw = rpy(3);

%control error is given by
error = rpy_desired-rpy;

% Relation between Tait-Bryan angles and angular velocities
%E_r = ...
E_r = [1 0 -sin(pitch); ...
       0 cos(roll) sin(roll)*cos(pitch);...
       0 -sin(roll) cos(roll)*cos(pitch)];

% rpy_dot = ... (from omega in body frame)
rpy_dot = E_r \ omega; %inv(E_r)*omega;

%control action U_2_3_4 is given by
%U_2_3_4 = ...

U_2_3_4 = diag(params.attitude_Kp)*error - diag(params.attitude_Kd)*rpy_dot;

== matlab function quadrotor/Subsystem3/Attitude dynamics/R to rpy ==
  data: R input; rpy output
function rpy = fcn(R)

%calculate roll pitch yaw from rotation matrix

[U,~,V] = svd(R);
R = U*V';

pitch = asin(-R(3,1));
roll = atan2(R(3,2), R(3,3));
yaw = atan2(R(2,1), R(1,1));

rpy = [roll; pitch; yaw];

== matlab function quadrotor/Subsystem3/Attitude dynamics/calculate_R_dot ==
  data: R input; R_dot output; omega input
function R_dot = fcn(R, omega)

%load parameters
params = parameters();

%normalize R every step to guarantee that R is orthogonal matrix (valid
%rotation)
[U,~,V] = svd(R);
R = U*V';

%Write R_dot = R*skew_omega
R_dot = R*[0 -omega(3) omega(2); omega(3) 0 -omega(1); -omega(2) omega(1) 0];

== matlab function quadrotor/Subsystem/Attitude dynamics/calculate_angular_acc ==
  data: omega_p input; angular_acc output; omega input
function angular_acc = fcn(omega_p, omega)
%omega_p is the rotational speed of the propellers. This vector must have
%size 4.
%omega is the angular velocity of the MAV expressed in body frame.

%load parameters
%Inertia is found under params.J
params = parameters();


U = params.allocation_matrix * (omega_p.^2);
angular_acc = params.J \ (-cross(omega, params.J * omega) + U(2:4));

== matlab function quadrotor/Subsystem3/Attitude dynamics/calculate_angular_acc ==
  data: omega_p input; angular_acc output; omega input
function angular_acc = fcn(omega_p, omega)
%omega_p is the rotational speed of the propellers. This vector must have
%size 4.
%omega is the angular velocity of the MAV expressed in body frame.

%load parameters
%Inertia is found under params.J
params = parameters();


U = params.allocation_matrix * (omega_p.^2);
angular_acc = params.J \ (-cross(omega, params.J * omega) + U(2:4));

== matlab function quadrotor/Subsystem3/Position controller/PD_position_controller_eqn ==
  data: p_d input; p input; rpy input; U_1 output; v input; roll_d output; pitch_d output
function [U_1, roll_d, pitch_d] = fcn(p_d, p, rpy, v)
%load parameters
%controller Kp is found under params.velocity_Kp
params = parameters();

%control error is given by
p_error = p_d - p;
v_error = zeros(3, 1) - v;
%control action U is given by
roll = rpy(1);
pitch = rpy(2);
yaw = rpy(3);

T = -diag(params.position_Kp) * p_error - diag(params.position_Kd) * v_error + [0; 0; params.m * params.g];

T_z = T(3);
U_1 = T_z / (cos(roll) * cos(pitch));
C_E1 = [cos(yaw) -sin(yaw) 0; sin(yaw) cos(yaw) 0; 0 0 1];
a = 1 / norm(T) * C_E1' * T;
roll_d = min(pi/6, max(-pi/6, -asin(a(2))));
pitch_d = min(pi/6, max(-pi/6, atan2(a(1), a(3))));

== matlab function quadrotor/Subsystem3/Translational dynamics/translational_dynamics_eqn ==
  data: R input; acc output; omega_p input
function acc = fcn(R, omega_p)

%load parameters
% to access for instance vehicle mass, use params.m.
% accelerational gravity is under params.g
params = parameters();

U = params.allocation_matrix*(omega_p.^2);

%acceleration is given by:
acc = - R * [0; 0; U(1)] / params.m + [0; 0; params.g];

== matlab function quadrotor/Subsystem/Translational dynamics/translational_dynamics_eqn ==
  data: R input; acc output; omega_p input
function acc = fcn(R, omega_p)

%load parameters
% to access for instance vehicle mass, use params.m.
% accelerational gravity is under params.g
params = parameters();

U = params.allocation_matrix*(omega_p.^2);

%acceleration is given by:
acc = - R * [0; 0; U(1)] / params.m + [0; 0; params.g];

== matlab function quadrotor/Subsystem/Attitude dynamics/calculate_R_dot ==
  data: R input; R_dot output; omega input
function R_dot = fcn(R, omega)

%load parameters
params = parameters();

%normalize R every step to guarantee that R is orthogonal matrix (valid
%rotation)
[U,~,V] = svd(R);
R = U*V';

%Write R_dot = R*skew_omega
R_dot = R*[0 -omega(3) omega(2); omega(3) 0 -omega(1); -omega(2) omega(1) 0];

== matlab function quadrotor/Subsystem/Attitude dynamics/R to rpy ==
  data: R input; rpy output
function rpy = fcn(R)

%calculate roll pitch yaw from rotation matrix

[U,~,V] = svd(R);
R = U*V';

pitch = asin(-R(3,1));
roll = atan2(R(3,2), R(3,3));
yaw = atan2(R(2,1), R(1,1));

rpy = [roll; pitch; yaw];

== matlab function quadrotor/Subsystem/Attitude PD controller/PD_attitude_controller_eqn ==
  data: rpy_desired input; U_2_3_4 output; rpy input; omega input
function U_2_3_4 = fcn(rpy_desired, rpy, omega)

%load parameters
%controller Kp is found under params.attitude_Kp
%controller Kd is found under params.attitude_Kd
params = parameters();

roll = rpy(1);
pitch = rpy(2);
yaw = rpy(3);

%control error is given by
error = rpy_desired-rpy;

% Relation between Tait-Bryan angles and angular velocities
%E_r = ...
E_r = [1 0 -sin(pitch); ...
       0 cos(roll) sin(roll)*cos(pitch);...
       0 -sin(roll) cos(roll)*cos(pitch)];

% rpy_dot = ... (from omega in body frame)
rpy_dot = E_r \ omega; %inv(E_r)*omega;

%control action U_2_3_4 is given by
%U_2_3_4 = ...

U_2_3_4 = diag(params.attitude_Kp)*error - diag(params.attitude_Kd)*rpy_dot;

== matlab function quadrotor/Subsystem1/Allocation/Control allocation ==
  data: U_1 input; omega_p output; U_2 input; U_3 input; U_4 input
function omega_p = fcn(U_1, U_2, U_3, U_4)

%load parameters

params = parameters();

omega_p_sqr = params.pinv_allocation_matrix*[U_1; U_2; U_3; U_4];

%make sure only positive values are allowed.
omega_p_sqr = max(omega_p_sqr, zeros(4,1));

%actual rotors velocities
omega_p = sqrt(omega_p_sqr);

== matlab function quadrotor/Subsystem/Allocation/Control allocation ==
  data: U_1 input; omega_p output; U_2 input; U_3 input; U_4 input
function omega_p = fcn(U_1, U_2, U_3, U_4)

%load parameters

params = parameters();

omega_p_sqr = params.pinv_allocation_matrix*[U_1; U_2; U_3; U_4];

%make sure only positive values are allowed.
omega_p_sqr = max(omega_p_sqr, zeros(4,1));

%actual rotors velocities
omega_p = sqrt(omega_p_sqr);

== matlab function quadrotor/Subsystem1/Attitude PD controller/PD_attitude_controller_eqn ==
  data: rpy_desired input; U_2_3_4 output; rpy input; omega input
function U_2_3_4 = fcn(rpy_desired, rpy, omega)

%load parameters
%controller Kp is found under params.attitude_Kp
%controller Kd is found under params.attitude_Kd
params = parameters();

roll = rpy(1);
pitch = rpy(2);
yaw = rpy(3);

%control error is given by
error = rpy_desired-rpy;

% Relation between Tait-Bryan angles and angular velocities
%E_r = ...
E_r = [1 0 -sin(pitch); ...
       0 cos(roll) sin(roll)*cos(pitch);...
       0 -sin(roll) cos(roll)*cos(pitch)];

% rpy_dot = ... (from omega in body frame)
rpy_dot = E_r \ omega; %inv(E_r)*omega;

%control action U_2_3_4 is given by
%U_2_3_4 = ...

U_2_3_4 = diag(params.attitude_Kp)*error - diag(params.attitude_Kd)*rpy_dot;

== matlab function quadrotor/Subsystem/Position controller/PD_position_controller_eqn ==
  data: p_d input; p input; rpy input; U_1 output; v input; roll_d output; pitch_d output
function [U_1, roll_d, pitch_d] = fcn(p_d, p, rpy, v)
%load parameters
%controller Kp is found under params.velocity_Kp
params = parameters();

%control error is given by
p_error = p_d - p;
v_error = zeros(3, 1) - v;
%control action U is given by
roll = rpy(1);
pitch = rpy(2);
yaw = rpy(3);

T = -diag(params.position_Kp) * p_error - diag(params.position_Kd) * v_error + [0; 0; params.m * params.g];

T_z = T(3);
U_1 = T_z / (cos(roll) * cos(pitch));
C_E1 = [cos(yaw) -sin(yaw) 0; sin(yaw) cos(yaw) 0; 0 0 1];
a = 1 / norm(T) * C_E1' * T;
roll_d = min(pi/6, max(-pi/6, -asin(a(2))));
pitch_d = min(pi/6, max(-pi/6, atan2(a(1), a(3))));
